simulink library "INT_IAirHt_DD"  (R2016b)
settings: Solver=VariableStepAuto  StartTime=0.0  StopTime=10.0  RelTol=1e-3
settings Model: Creator=liutao  LastModifiedBy=liutao

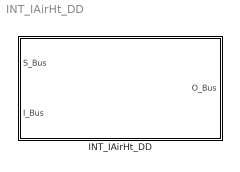
== system INT_IAirHt_DD ==
  INT_IAirHt_DD : Subsystem

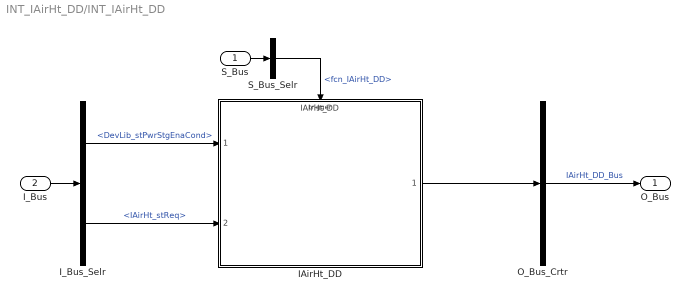
== system INT_IAirHt_DD/INT_IAirHt_DD ==
  S_Bus : Inport
  I_Bus : Inport  Port=2
  IAirHt_DD : ModelReference  ModelNameDialog=IAirHt_DD  SimulationMode=Normal  ModelReferenceVersion=1.17  TriggerPortName=function  TriggerPortTriggerType=function-call  TriggerPortStatesWhenEnabling=held
  I_Bus_Selr : BusSelector  OutputSignals=DevLib_stPwrStgEnaCond,IAirHt_stReq
  O_Bus_Crtr : BusCreator  Inputs=1
  S_Bus_Selr : BusSelector  OutputSignals=fcn_IAirHt_DD
  O_Bus : Outport
  wires:
  S_Bus_Selr/1 -> IAirHt_DD/Trigger  "<fcn_IAirHt_DD>"
  S_Bus/1 -> S_Bus_Selr/1
  I_Bus/1 -> I_Bus_Selr/1
  I_Bus_Selr/1 -> IAirHt_DD/1  "<DevLib_stPwrStgEnaCond>"
  I_Bus_Selr/2 -> IAirHt_DD/2  "<IAirHt_stReq>"
  O_Bus_Crtr/1 -> O_Bus/1  "IAirHt_DD_Bus"
  IAirHt_DD/1 -> O_Bus_Crtr/1
